simulink model "ContributionFlow"  (R2023b)
settings: Solver=FixedStepDiscrete  StartTime=0.0  StopTime=2035-year(now)  RelTol=1e-3  EnableMultiTasking=on
PreLoadFcn:
  | % K goes from 0 (all to roth) to 1 (all to deferred)
  | k=17/19;
StopFcn:
  | Cash    = xFinal.loggedStates(1).values + ... % after tax
  |               xFinal.loggedStates(3).values;      % roth
  | 
  | Taxable = xFinal.loggedStates(4).values + ... % hsa
  |                xFinal.loggedStates(2).values + ... % deferred
  |               xFinal.loggedStates(15).values + ... % tiaa
  |               xFinal.loggedStates(17).values;      % company match
  | 
  | Taxes = xFinal.loggedStates(7).values; % cumulative taxes
  | 
  | % Note that technically the after tax account growth
  | % is taxable (only the growth), however it's not taxable
  | % anymore if one moves the amount to roth, so in
  | % the above the after tax voluntary contribution amount
  | % is connsidered fully non taxable
libraries: moneylib x10
settings Model: Creator=gcampa  LastModifiedBy=gcampa
settings SolverCC: AlgebraicLoopSolver=TrustRegion
settings DataIOCC: LimitDataPoints=on  SaveFinalState=on  SaveOperatingPoint=on  SaveFormat=Array  SaveOutput=off  SignalLogging=off  DSMLogging=off  SaveTime=off  ReturnWorkspaceOutputs=off
settings OptimizationCC: ReuseModelBlockBuffer=off  LifeSpan=inf
settings DebuggingCC: UnderspecifiedInitializationDetection=Classic  MergeDetectMultiDrivingBlocksExec=none  SolverPrmCheckMsg=warning  FcnCallInpInsideContextMsg=warning  UnconnectedInputMsg=warning  UnconnectedOutputMsg=warning  UnconnectedLineMsg=warning  StateNameClashWarn=warning  SFUnexpectedBacktrackingDiag=warning  SFNoUnconditionalDefaultTransitionDiag=warning  SFExecutionAtInitializationDiag=none  ArithmeticOperatorsInVariantConditions=warning
settings HardwareCC: ProdBitPerPointer=32  ProdBitPerSizeT=32  ProdBitPerPtrDiffT=32  ProdLargestAtomicFloat=None  ProdIntDivRoundTo=Undefined  ProdEndianess=Unspecified  ProdWordSize=32  ProdHWDeviceType=32-bit Generic
settings ModelReferenceCC: EnableRefExpFcnMdlSchedulingChecks=on  PropagateSignalLabelsOutOfModel=off
settings SFSimCC: SimUseLocalCustomCode=off  CustomCodeUndefinedFunction=UseInterfaceOnly
settings RTWCC: RTWUseLocalCustomCode=off  DLArmComputeVersion=19.05
settings CodeAppCC: StateflowObjectComments=on
settings GRTTargetCC: TargetLangStandard=C89/C90 (ANSI)
settings ConfigComp: CovMetricSettings=dw  CovSaveCumulativeToWorkspaceVar=on  CovSaveSingleToWorkspaceVar=on  CovExternalEMLEnable=off  CovSFcnEnable=off

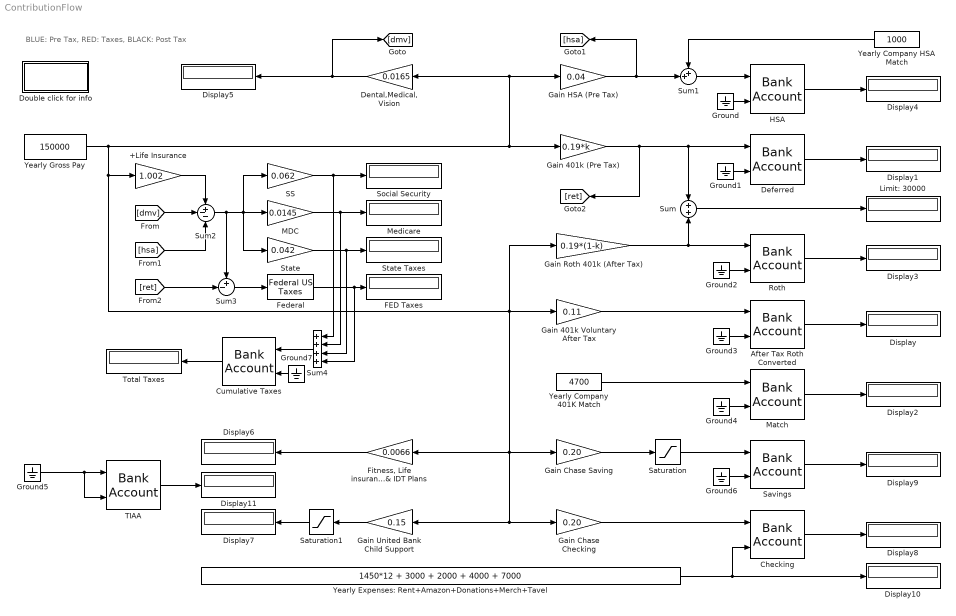
== system ContributionFlow ==
  note: BLUE: Pre Tax, RED: Taxes, BLACK: Post Tax
  +Life Insurance : Gain  Gain=1.002
  After Tax Roth Converted : moneylib/Bank Account  i=0.03  j=0.02  x0=35000
  Checking : moneylib/Bank Account  i=0.03  j=0.02  x0=11000
  Cumulative Taxes : moneylib/Bank Account  i=0  j=0  x0=0
  Deferred : moneylib/Bank Account  i=0.03  j=0.02  x0=300000
  "Dental,Medical, Vision" : Gain  Gain=0.0165
  Display{,1..11} (12 alike) : Display
      settings: Format=bank
  Double click for info : Subsystem
      mask Display: disp('Explanation')
  FED Taxes : Display
      settings: Format=bank
  Federal : moneylib/Federal US Taxes  x=[9875 40125 85525 163300 207350 518400]  p=[0.10 0.12 0.22 0.24 0.32 0.35 0.37]
  "Fitness, Life insurance Legal & IDT Plans" : Gain  Gain=0.0066
  Gain 401k (Pre Tax) : Gain  Gain=0.19*k
  Gain 401k Voluntary After Tax : Gain  Gain=0.11
  Gain Chase Checking : Gain  Gain=0.20
  Gain Chase Saving : Gain  Gain=0.20
  Gain HSA (Pre Tax) : Gain  Gain=0.04
  Gain Roth 401k (After Tax) : Gain  Gain=0.19*(1-k)
  Gain United Bank Child Support : Gain  Gain=0.15
  Ground{,1..7} (8 alike) : Ground
  HSA : moneylib/Bank Account  i=0.03  j=0.02  x0=20000
  Limit: 30000 : Display
      settings: Format=bank
  MDC : Gain  Gain=0.0145
  Match : moneylib/Bank Account  i=0.03  j=0.02  x0=150000
  Medicare : Display
      settings: Format=bank
  Roth : moneylib/Bank Account  i=0.03  j=0.02  x0=220000
  SS : Gain  Gain=0.062
  Saturation : Saturate  UpperLimit=1000*(26+4)
  Saturation1 : Saturate  UpperLimit=785*26  LowerLimit=785*26
  Savings : moneylib/Bank Account  i=0.03  j=0.02  x0=15000
  Social Security : Display
      settings: Format=bank
  State : Gain  Gain=0.042
  State Taxes : Display
      settings: Format=bank
  Sum : Sum  Inputs=+|+
  Sum1 : Sum  Inputs=++|
  Sum2 : Sum  Inputs=+--
  Sum3 : Sum  Inputs=+-|
  Sum4 : Sum  Inputs=4
  TIAA : moneylib/Bank Account  i=0.03  j=0.00  x0=128873
  Total Taxes : Display
      settings: Format=bank
  Yearly Company 401K Match : Constant  Value=4700
  Yearly Company HSA Match : Constant  Value=1000
  "Yearly Expenses: Rent+Amazon+Donations+Merch+Tavel " : Constant  Value=1450*12 + 3000 + 2000 + 4000 + 7000
  Yearly Gross Pay : Constant  Value=150000
  wires:
  After Tax Roth Converted/1 -> Display/1
  Gain 401k Voluntary After Tax/1 -> After Tax Roth Converted/1
  Ground3/1 -> After Tax Roth Converted/2
  Ground1/1 -> Deferred/2
  Gain 401k (Pre Tax)/1 -> [ret], Deferred/1, Sum/1
  Deferred/1 -> Display1/1
  Match/1 -> Display2/1
  Yearly Company 401K Match/1 -> Match/1
  Ground4/1 -> Match/2
  Ground2/1 -> Roth/2
  Gain Roth 401k (After Tax)/1 -> Roth/1, Sum/2
  Roth/1 -> Display3/1
  Federal/1 -> FED Taxes/1, Sum4/4
  State/1 -> Sum4/3, State Taxes/1
  SS/1 -> Social Security/1, Sum4/1
  MDC/1 -> Sum4/2, Medicare/1
  Yearly Gross Pay/1 -> Gain 401k (Pre Tax)/1, "Dental,Medical, Vision"/1, Gain HSA (Pre Tax)/1, +Life Insurance/1, "Fitness, Life insurance Legal & IDT Plans"/1, Gain Chase Checking/1, Gain United Bank Child Support/1, Gain Chase Saving/1, Gain 401k Voluntary After Tax/1, Gain Roth 401k (After Tax)/1
  Sum/1 -> Limit: 30000/1
  Ground/1 -> HSA/2
  HSA/1 -> Display4/1
  "Dental,Medical, Vision"/1 -> [dmv], Display5/1
  "Fitness, Life insurance Legal & IDT Plans"/1 -> Display6/1
  Gain HSA (Pre Tax)/1 -> [hsa], Sum1/2
  Sum1/1 -> HSA/1
  Yearly Company HSA Match/1 -> Sum1/1
  Gain United Bank Child Support/1 -> Saturation1/1
  Gain Chase Checking/1 -> Checking/1
  Checking/1 -> Display8/1
  "Yearly Expenses: Rent+Amazon+Donations+Merch+Tavel "/1 -> Checking/2, Display10/1
  Gain Chase Saving/1 -> Saturation/1
  Savings/1 -> Display9/1
  Ground6/1 -> Savings/2
  Saturation/1 -> Savings/1
  Saturation1/1 -> Display7/1
  Ground5/1 -> TIAA/1, TIAA/2
  TIAA/1 -> Display11/1
  Sum2/1 -> Sum3/1, State/1, SS/1, MDC/1
  [ret] -> Sum3/2
  Sum3/1 -> Federal/1
  [hsa] -> Sum2/3
  [dmv] -> Sum2/2
  +Life Insurance/1 -> Sum2/1
  Sum4/1 -> Cumulative Taxes/1
  Cumulative Taxes/1 -> Total Taxes/1
  Ground7/1 -> Cumulative Taxes/2

== system ContributionFlow/Double click for info ==
  note: This simulation shows how an annual income flows from the paycheck into several banking and investment accounts, over a contribution period of 35 years. The blue blocks handle pre-tax income, the red one handle taxex, and the black ones handle post-tax income.
      |
      | The yearly income is assumed constant and equal to 150K$, (though in reality it would increase over time). About 25% of income is used for taxes and the remaining 75% gets distributed to various destinations (4% in a tax deferred HSA, 17% to tax deferred 401K, 2% to a Roth 401K, 20% to a savings account, and 20% to a checking account, plus a small amount in pre-tax medical expenses). Retirement accounts earn an interest rate of 3% at the end of each year, while savings and checking accounts do not earn interest (see the account mask parameters). Note that a parameter k that is loaded by a PreLoadFcn (see Model Settings -> Model Properties -> Callbacks -> PreLoadFcn) regulates the inflow of tax-deferred vs roth accounts (k=0 means 19% goes to tax deferred 401K and 0% to Roth 401k, k=1 all 19% goes to Roth).
      |
      | Inflation is set to 2% at year (see the account blocks mask parameters), but it has an effect only on the Checking account, (because is the only one with nonzero expenses), specifically causing the expense withdrawals to increase progressively each year. Note that the 401K account and the 401K Roth one start with 50K$ and 10K% respectively, at the beginning of the simulation.
      |
      | At the end of the simulation, a stop function callback (see Model Settings -> Model Properties -> Callbacks -> StopFcn) saves in the workspace variable "Cash" the total amounts of money in non-taxable accounts, such as Roth, Savings and Chacking. It also saves in the workspace variable "Taxable" the total amounts of money in taxable accounts such as 401K and HSA (conservatively assuming that HSA modey are not used for medical expenses). These two workspace variables can then be used in the "DistributionFlow.mdl" simulation, which shows how both non-taxable and taxable money (together with social security) are distributed for retirement expenses.
